simulink model "PI_Controller"  (R2020b)
settings: Solver=VariableStepAuto  StartTime=0.0  StopTime=10.0  RelTol=1e-3
values from neighbouring files (symbols this model uses):
  Ki = 40.0    [cruisecontrol_para.sldd]
  Kp = 800.0    [cruisecontrol_para.sldd]
settings Model: Creator=shivanshu shukla  LastModifiedBy=shivanshu shukla
settings DataIOCC: SaveOutput=off  SaveTime=off

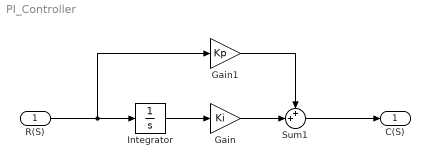
== system PI_Controller ==
  R(S) : Inport  OutDataTypeStr=double  PortDimensions=1  SampleTime=0
  Gain : Gain  Gain=Ki
  Gain1 : Gain  Gain=Kp
  Integrator : Integrator
  Sum1 : Sum  Inputs=++|
  C(S) : Outport  OutDataTypeStr=double  PortDimensions=1  SampleTime=0
  wires:
  Gain1/1 -> Sum1/1
  R(S)/1 -> Gain1/1, Integrator/1
  Sum1/1 -> C(S)/1
  Gain/1 -> Sum1/2
  Integrator/1 -> Gain/1
